simulink model "STV_Polytope_test"  (Simulink 7.3)
settings: Solver=ode45  StartTime=0.0  StopTime=10.0  RelTol=1e-3
settings Model: Creator=MD710  LastModifiedBy=MD710
settings DebuggingCC: SaveWithParameterizedLinksMsg=none  SolverPrmCheckMsg=none  MultiTaskDSMMsg=warning  MultiTaskCondExecSysMsg=none  FcnCallInpInsideContextMsg=Enable All  StrictBusMsg=None
settings HardwareCC: TargetHWDeviceType=32-bit Generic
settings RTWCC: IncludeERTFirstTime=on
settings GRTTargetCC: TargetFcnLib=ansi_tfl_tmw.mat

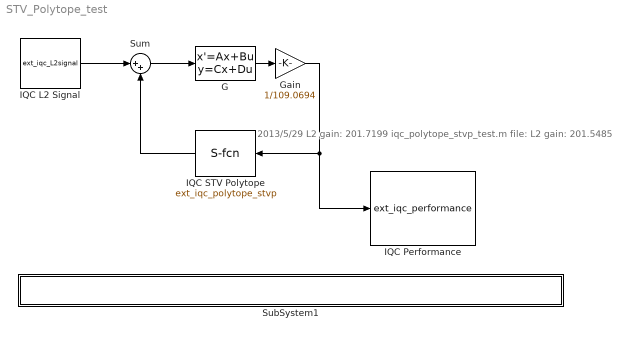
== system STV_Polytope_test ==
  note: 2013/5/29 L2 gain: 201.7199
      | iqc_polytope_stvp_test.m file:
      | L2 gain: 201.5485
  G : StateSpace  A=|  B=|  C=|  D=[0 0;0 0]
      A=|
      | [-1.4928 -0.9898 1.1380 -0.3306;
      |     -0.6451 -0.1645 -0.6841 -0.8436;
      |     0.8057 0.2895 -2.7960 0.4978;
      |     0.2316 1.4789 -0.0729 -0.0156]
      B=|
      | [-0.5465 -0.8542;
      |     -0.8468 -1.2013;
      |     -0.2463   -0.1199;
      |      0.6630   -0.0653]
      C=|
      | [0.4853 -0.1497 -0.0793 -0.6065;
      |     -0.5955 -0.4348 1.5352 -1.347]
  Gain : Gain  Gain=1/109.0694
  IQC L2 Signal : M-S-Function  FunctionName=ext_iqc_L2signal  Parameters=sig_size,sam_time,sig_type,tru_time,sig_amp,sig_fre,user_cus  mask(IQC L2 signal(ver:0.1)){sig_size=2, sam_time=0, sig_type=Step, tru_time=10, sig_amp=1, sig_fre=1, user_cus='2*exp(3*t)'}
      mask prompts: sig_size "Signal Dimension:(Default: 1)"; sam_time "Sample Time:(Default: 0)"; sig_type "Signal Type:"; tru_time "Truncation Time:"; sig_amp "Maximum Amplitude:"; sig_fre "Frequency:"; user_cus "Custom:"
      mask help:
      | Important:
      | In IQC procedure step (as commond iqc_gain_tbx, the task is get
      | L2 gain value), regardless of the user to choose which option (ex sine...),
      | here regarded as generalized L2 signal.
      mask StyleString: edit,edit,popup(Step|Square wave|Sine wave|Custom|Random|External),edit,edit,edit,edit
      mask CallbackString: ||iqc_block_cho(gcb,'L2signal_type')||||
      mask TabNameString: Generalized Parameters,Generalized Parameters,Simulink Parameters,Simulink Parameters,Simulink Parameters,Simulink Parameters,Simulink Parameters
      mask Display: plot(0:0.1:10,[sin(0:0.1:6.2) zeros(1,38)])
  IQC Performance : M-S-Function  FunctionName=ext_iqc_performance  Parameters=imp_met,save_lin_com,isiqcbode,fre_ran,uselmitool,lmi_par  mask(IQC Performance(ver:0.1)){imp_met=Only Calculation, save_lin_com=off, isiqcbode=off, fre_ran='', uselmitool=lmilab, lmi_par=''}
      mask prompts: imp_met "Implementation Methods"; save_lin_com "Save the Linear File and Command File"; isiqcbode "Display IQC Bode Figure"; fre_ran "Frequency Range:(Default: empty)"; uselmitool "LMI Tool:"; lmi_par "Parameter:(if empty use define)"
      mask help:
      | Important:
      | In IQC toolbox calculate step (as commond iqc_gain_tbx, the task is get
      | L2 gain value), regardless of the user to connect any signal input(Even if
      | not a signal), here regarded as generalized L2 signal.
      |
      | Example 1: setlmioptions('',[0 200 0 0 777])
      | the block parameter is
      | LMI Tool: lmilab
      | Parameter:
      |        [0 200 0 0 777]
      |
      | Example 2: setlmioptions('yalmip','solver','sdpt3','verbose',1)
      | the block parameter is
      | LMI Tool: yalmip
      | Parameter:
      |        {'solver',sdpt3','verbose',1}
      mask Help:
      | <a href="matlab:doc abst_init_iqc;">abst_init_iqc</a>
      | <a href="matlab:doc setlmioptions;">setlmioptions</a>
      | <a href="matlab:doc iqc_gain_tbx;">iqc_gain_tbx</a>
      mask StyleString: popup(Calculation and Simulation|Only Calculation|Only Simulation),checkbox,checkbox,edit,popup(lmilab|yalmip),edit
      mask CallbackString: iqc_block_cho(gcb,'performance_imp')||iqc_block_cho(gcb,'performance_bodefre')|||
      mask TabNameString: Parameter,Parameter,Parameter,Parameter,LMI Parameter,LMI Parameter
      mask Display: fprintf('In -> Out \n performance \n L2 gain:\n%4.4f',201.4738);
  IQC STV Polytope : M-S-Function  FunctionName=ext_iqc_polytope_stvp  Parameters=arr_del,arr_ddel,str_mat,out_var  mask(IQC STV Polytope(ver:0.1)){arr_del={1.96*[1 0;0 1],1.96*[1 0;0 -1],1.96*[-1 0;0 0],1.96*[-1 0;0 -1]}, arr_ddel={[0.1 0;0 0.1],[0.1 0;0 -0.1],[-0.1 0;0 0.1],[-0.1 0;0 -0.1]}, str_mat=[1 0;0 2], out_var=''}
      mask prompts: arr_del "Cell Array for delta:"; arr_ddel "Cell Array for d(delta)/dt:"; str_mat "LMI-Lab Structure Matrix:"; out_var "Output Variable:(Default: empty)"
      mask help:
      | Example: [w,X,Y,Z,Lambda]=iqc_polytope_stvp(v,C1,C2,Lambdastruc);
      | Cell Array for delta:
      |              C1
      | Cell Array for d(delta)/dt
      |              C2
      | LMI-Lab Structure Matrix:
      |          Lambdastruc
      | Output Variable:
      |        {'X','Y','Z','Lambda'}
      mask Help: eval('doc iqc_polytope_stvp')
      mask Display: disp('STV\nPolytopic');
  SubSystem1 : Subsystem  mask{filename=iqc_polytope_stvp_test.m}
      mask init:
      | x_dir=which(filename);
      | x=x_dir;
      settings: OpenFcn=|
      | x_dir=which('iqc_polytope_stvp_test.m');
      | x=x_dir;
      | edit(x);
      mask Display: disp(['MATLAB file: ' x]);
  Sum : Sum  Inputs=|++
  wires:
  IQC L2 Signal/1 -> Sum/1
  Sum/1 -> G/1
  IQC STV Polytope/1 -> Sum/2
  G/1 -> Gain/1
  Gain/1 -> IQC Performance/1, IQC STV Polytope/1

== system STV_Polytope_test/SubSystem1 ==
